simulink model "rlWatertankPITuningUseCase1"  (R2026a)
settings: Solver=ode45  StopTime=Tf  EnableMultiTasking=on
values from neighbouring files (symbols this model uses):
  Ts = 1    [DA2_main.m]    (also in LSTMController.m; TunePIControllerWithReinforcementLearningExample.m; build_compare_model.m)
undefined symbols (not defined in the file or in its folder): DiscIntNeverNeededParam
libraries: simulink x1, rllib x1
settings Model: Creator=The MathWorks, Inc.  LastModifiedBy=The MathWorks, Inc.
settings DataIOCC: SignalLoggingName=logsOut
settings OptimizationCC: InitFltsAndDblsToZero=on
settings DebuggingCC: SaveWithParameterizedLinksMsg=none  SignalResolutionControl=TryResolveAllWithWarning  MultiTaskDSMMsg=warning
settings HardwareCC: ProdHWDeviceType=Specified
settings GRTTargetCC: TargetFcnLib=ansi_tfl_tmw.mat  CombineOutputUpdateFcns=off  GRTInterface=on

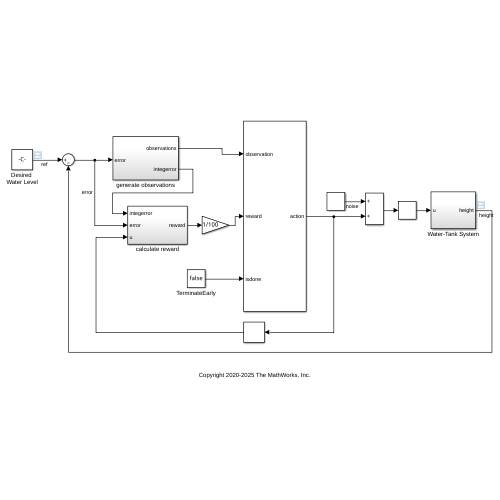
[thumbnail: Simulink's stored preview of the top-level diagram]
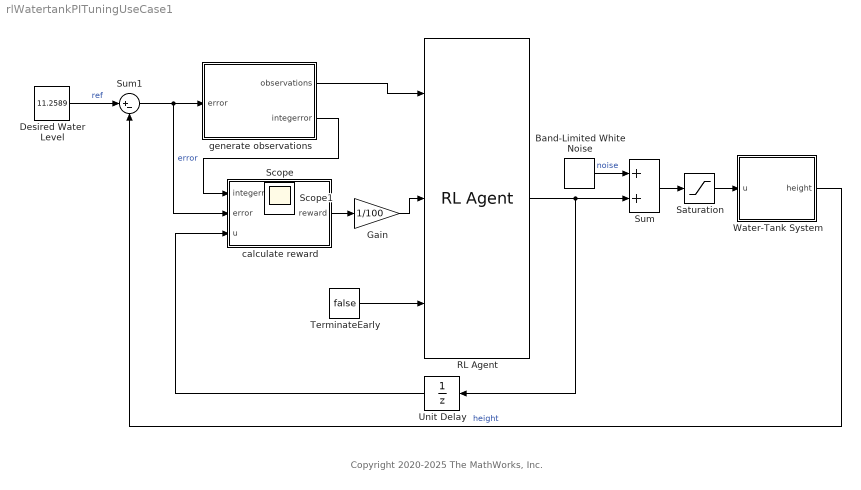
== system rlWatertankPITuningUseCase1 ==
  note: Copyright 2020-2025 The MathWorks, Inc.
  Band-Limited White Noise : simulink/Sources/Band-Limited White Noise  Cov=0.01  Ts=1  seed=[23341]
  Desired Water Level : Constant  Value=11.2589
  Gain : Gain  Gain=1/100
  RL Agent : rllib/RL Agent  Agent=agent1  ExternalActionAsInput=off  ProvideLastAction=off  ProvideCumRwd=off  TreatAsDirectFeedthrough=on  UseStrictObservationDataTypes=off
  Saturation : Saturate  UpperLimit=12  LowerLimit=0
  Sum : Sum
  Sum1 : Sum  Inputs=|+-  SaturateOnIntegerOverflow=on
  TerminateEarly : Constant  Value=false
  Unit Delay : UnitDelay  SampleTime=-1
  Water-Tank System : Subsystem
  calculate reward : Subsystem
  generate observations : Subsystem
  Scope : Scope
      settings: ActiveDisplayYMinimum=0.26116  ActiveDisplayYMaximum=2.71198
  Scope1 : Scope
  wires:
  Desired Water Level/1 -> Sum1/1  "ref"
  Sum1/1 -> calculate reward/2(error), generate observations/1(error)  "error"
  generate observations/1(observations) -> RL Agent/1
  Water-Tank System/1(height) -> Sum1/2  "height"
  Unit Delay/1 -> calculate reward/3(u)
  calculate reward/1(reward) -> Gain/1
  TerminateEarly/1 -> RL Agent/3
  Gain/1 -> RL Agent/2
  RL Agent/1 -> Unit Delay/1, Sum/2
  Saturation/1 -> Water-Tank System/1(u)
  Band-Limited White Noise/1 -> Sum/1  "noise"
  Sum/1 -> Saturation/1
  generate observations/2(integerror) -> calculate reward/1(integerror)

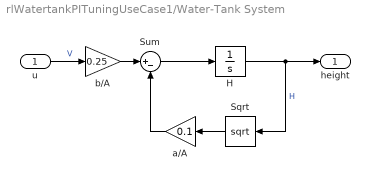
== system rlWatertankPITuningUseCase1/Water-Tank System ==
  u : Inport
  H : Integrator  InitialCondition=10.2886  LimitOutput=on  LowerSaturationLimit=0
  Sqrt : Sqrt  OutputSignalType=real
  Sum : Sum  Inputs=|+-  SaturateOnIntegerOverflow=on
  a/A : Gain  Gain=0.1  SaturateOnIntegerOverflow=on  OutDataTypeStr=Inherit: Same as input  ParamDataTypeStr=Inherit: Same as input
  b/A : Gain  Gain=0.25  SaturateOnIntegerOverflow=on  OutDataTypeStr=Inherit: Same as input  ParamDataTypeStr=Inherit: Same as input
  height : Outport  VectorParamsAs1DForOutWhenUnconnected=off
  wires:
  b/A/1 -> Sum/1
  Sum/1 -> H/1
  H/1 -> Sqrt/1, height/1  "H"
  Sqrt/1 -> a/A/1
  a/A/1 -> Sum/2
  u/1 -> b/A/1  "V"

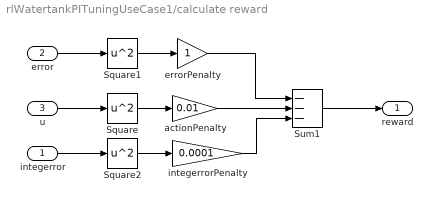
== system rlWatertankPITuningUseCase1/calculate reward ==
  integerror : Inport
  error : Inport  Port=2
  u : Inport  Port=3
  Square : Math  Operator=square
  Square1 : Math  Operator=square
  Square2 : Math  Operator=square
  Sum1 : Sum  Inputs=---  OutDataTypeStr=double
  actionPenalty : Gain  Gain=0.01
  errorPenalty : Gain
  integerrorPenalty : Gain  Gain=0.0001
  reward : Outport  VectorParamsAs1DForOutWhenUnconnected=off
  wires:
  Square1/1 -> errorPenalty/1
  errorPenalty/1 -> Sum1/1
  actionPenalty/1 -> Sum1/2
  Square/1 -> actionPenalty/1
  u/1 -> Square/1
  error/1 -> Square1/1
  Sum1/1 -> reward/1
  integerror/1 -> Square2/1
  integerrorPenalty/1 -> Sum1/3
  Square2/1 -> integerrorPenalty/1

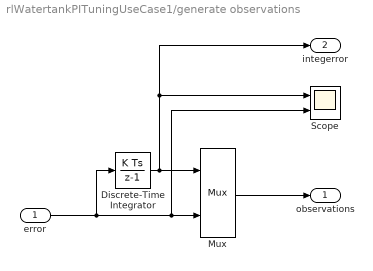
== system rlWatertankPITuningUseCase1/generate observations ==
  error : Inport
  Discrete-Time Integrator : DiscreteIntegrator  SampleTime=Ts  ICPrevOutput=DiscIntNeverNeededParam  ICPrevScaledInput=DiscIntNeverNeededParam
  Mux : Mux  Inputs=2
  Scope : Scope  NumInputPorts=2
      settings: TimeSpan=100  ActiveDisplayYMinimum=-3  ActiveDisplayYMaximum=12  DataLoggingVariableName=ScopeData2
  observations : Outport  VectorParamsAs1DForOutWhenUnconnected=off
  integerror : Outport  Port=2  VectorParamsAs1DForOutWhenUnconnected=off
  wires:
  Discrete-Time Integrator/1 -> integerror/1, Scope/1, Mux/1
  error/1 -> Discrete-Time Integrator/1, Scope/2, Mux/2
  Mux/1 -> observations/1
